simulink model "DIPCtranslation"  (R2014b)
settings: Solver=ode45  StartTime=0.0  StopTime=3.0  RelTol=1e-3
values from neighbouring files (symbols this model uses):
  deltav = 2000    [DIPCinit.m]
  ds = 0    [DIPCinit.m]
  dv = 5000    [DIPCinit.m]
  g = [0;0;0]    [DIPCinit.m]
  j0 = 1    [DIPCinit.m]
  j1 = 10    [DIPCinit.m]
  j2 = 10    [DIPCinit.m]
  j3 = 10    [DIPCinit.m]
  j4 = 10    [DIPCinit.m]
  jv = 1    [DIPCinit.m]
  kappav = 2000    [DIPCinit.m]
  ks = 3000    [DIPCinit.m]
  kv = 20000    [DIPCinit.m]
  m0 = 10    [DIPCinit.m]
  m1 = 10    [DIPCinit.m]
  m2 = 10    [DIPCinit.m]
  m3 = 10    [DIPCinit.m]
  m4 = 10    [DIPCinit.m]
  mv = 10    [DIPCinit.m]
libraries: aerolibutil x3, dspinverses x2, aerolibtransform2 x1, simulink x1
settings Model: Creator=Martin  LastModifiedBy=Martin

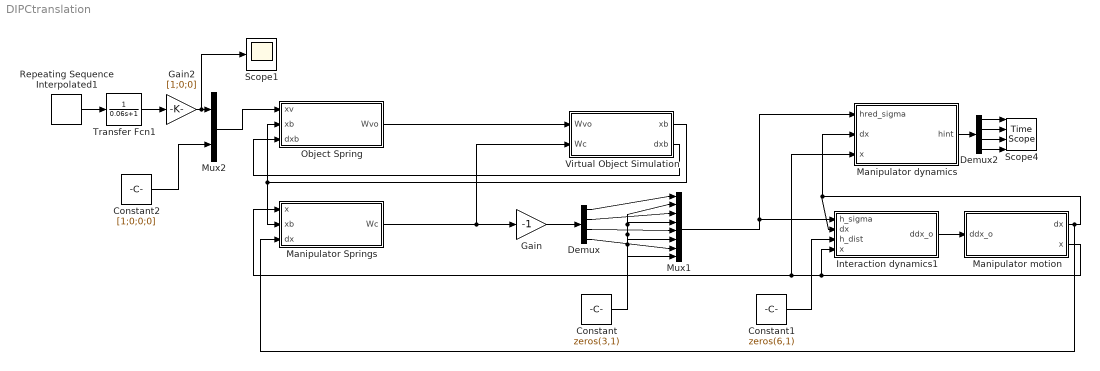
== system DIPCtranslation ==
  Constant : Constant  Value=zeros(3,1)
  Constant1 : Constant  Value=zeros(6,1)
  Constant2 : Constant  Value=[1;0;0;0]
  Demux : Demux
  Demux2 : Demux
  Gain : Gain  Gain=-1
  Gain2 : Gain  Gain=[1;0;0]
  Interaction dynamics1 : Subsystem
  Manipulator Springs : Subsystem
  Manipulator dynamics : Subsystem
  Manipulator motion : Subsystem
  Mux1 : Mux  Inputs=8
  Mux2 : Mux  Inputs=2
  Object Spring : Subsystem
  Repeating Sequence Interpolated1 : simulink/Sources/Repeating Sequence Interpolated  OutValues=[0 0 2 2 4 4 -2 -2 0 0].'  TimeValues=[0 0.1 0.14 0.9 0.96 1.8 1.95 2.4 2.6 3].'  LookUpMeth=Interpolation-Use End Values  tsamp=0.01  OutMin=[]  OutMax=[]  OutDataTypeStr=double  OutputDataTypeScalingMode=double  OutDataType=fixdt(0,8)  OutScaling=2^-10
  Scope1 : Scope
      settings: SaveName=ScopeData8
  Scope4 : TimeScope  NumInputPorts=4
  Transfer Fcn1 : TransferFcn  Denominator=[0.06 1]
  Virtual Object Simulation : Subsystem
  wires:
  Object Spring/1(Wvo) -> Virtual Object Simulation/1(Wvo)
  Virtual Object Simulation/1(xb) -> Object Spring/2(xb), Manipulator Springs/2(xb)
  Manipulator Springs/1(Wc) -> Gain/1, Virtual Object Simulation/2(Wc)
  Interaction dynamics1/1(ddx_o) -> Manipulator motion/1(ddx_o)
  Gain/1 -> Demux/1
  Demux/1 -> Mux1/1
  Demux/2 -> Mux1/3
  Constant/1 -> Mux1/8, Mux1/6, Mux1/4, Mux1/2
  Constant1/1 -> Interaction dynamics1/3(h_dist)
  Mux1/1 -> Manipulator dynamics/1(hred_sigma), Interaction dynamics1/1(h_sigma)
  Manipulator motion/1(dx) -> Manipulator Springs/3(dx), Manipulator dynamics/2(dx), Interaction dynamics1/2(dx)
  Manipulator motion/2(x) -> Manipulator dynamics/3(x), Manipulator Springs/1(x), Interaction dynamics1/4(x)
  Virtual Object Simulation/2(dxb) -> Object Spring/3(dxb)
  Demux/3 -> Mux1/5
  Demux/4 -> Mux1/7
  Manipulator dynamics/1(hint) -> Demux2/1
  Demux2/2 -> Scope4/2
  Demux2/4 -> Scope4/4
  Demux2/3 -> Scope4/3
  Demux2/1 -> Scope4/1
  Repeating Sequence Interpolated1/1 -> Transfer Fcn1/1
  Transfer Fcn1/1 -> Gain2/1
  Gain2/1 -> Scope1/1, Mux2/1
  Mux2/1 -> Object Spring/1(xv)
  Constant2/1 -> Mux2/2

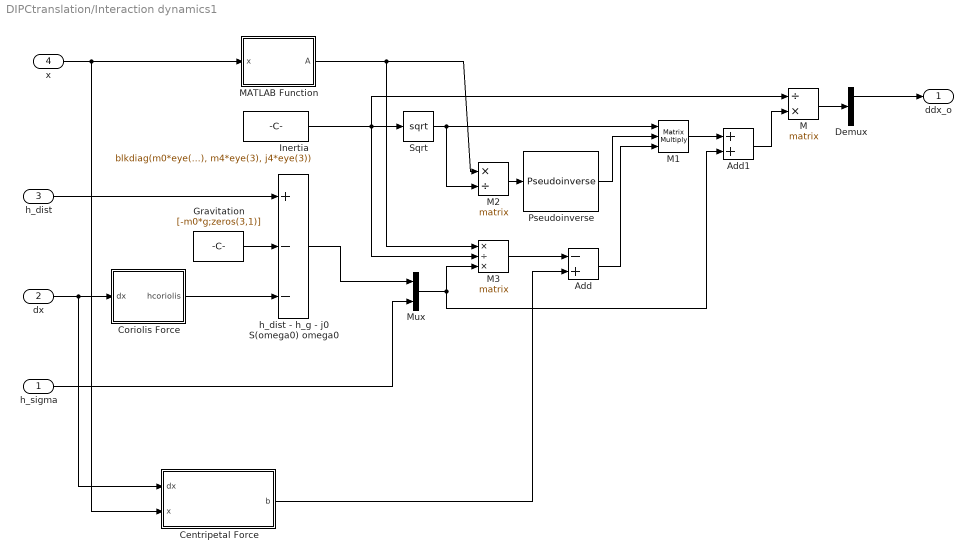
== system DIPCtranslation/Interaction dynamics1 ==
  h_sigma : Inport
  dx : Inport  Port=2
  h_dist : Inport  Port=3
  x : Inport  Port=4
  Add : Sum  Inputs=-+
  Add1 : Sum
  Centripetal Force : MATLAB Function  TreatAsAtomicUnit=on
  Coriolis Force : MATLAB Function  TreatAsAtomicUnit=on
  Demux : Demux  Outputs=5
  Gravitation : Constant  Value=[-m0*g;zeros(3,1)]
  Inertia : Constant  Value=blkdiag(m0*eye(3),j0*eye(3),m1*eye(3), j1*eye(3), m2*eye(3), j2*eye(3),m3*eye(3), j3*eye(3), m4*eye(3), j4*eye(3))
  M : Product  Inputs=/*  Multiplication=Matrix(*)
  M1 : Product  Inputs=***  Multiplication=Matrix(*)
  M2 : Product  Inputs=*/  Multiplication=Matrix(*)
  M3 : Product  Inputs=*/*  Multiplication=Matrix(*)
  MATLAB Function : MATLAB Function  TreatAsAtomicUnit=on
  Mux : Mux  Inputs=2
  Pseudoinverse : dspinverses/Pseudoinverse  wanterr=off
  Sqrt : Sqrt  SaturateOnIntegerOverflow=on
  "h_dist - h_g - j0 S(omega0) omega0 " : Sum  Inputs=+--
  ddx_o : Outport
  wires:
  h_dist/1 -> "h_dist - h_g - j0 S(omega0) omega0 "/1
  Gravitation/1 -> "h_dist - h_g - j0 S(omega0) omega0 "/2
  dx/1 -> Centripetal Force/1(dx), Coriolis Force/1(dx)
  Coriolis Force/1(hcoriolis) -> "h_dist - h_g - j0 S(omega0) omega0 "/3
  x/1 -> MATLAB Function/1(x), Centripetal Force/2(x)
  Inertia/1 -> M/1, M3/2, Sqrt/1
  Sqrt/1 -> M2/2, M1/1
  MATLAB Function/1(A) -> M3/1, M2/1
  M2/1 -> Pseudoinverse/1
  Pseudoinverse/1 -> M1/2
  Add/1 -> M1/3
  Centripetal Force/1(b) -> Add/2
  M3/1 -> Add/1
  Mux/1 -> Add1/2, M3/3
  "h_dist - h_g - j0 S(omega0) omega0 "/1 -> Mux/1
  h_sigma/1 -> Mux/2
  M/1 -> Demux/1
  Demux/1 -> ddx_o/1
  M1/1 -> Add1/1
  Add1/1 -> M/2

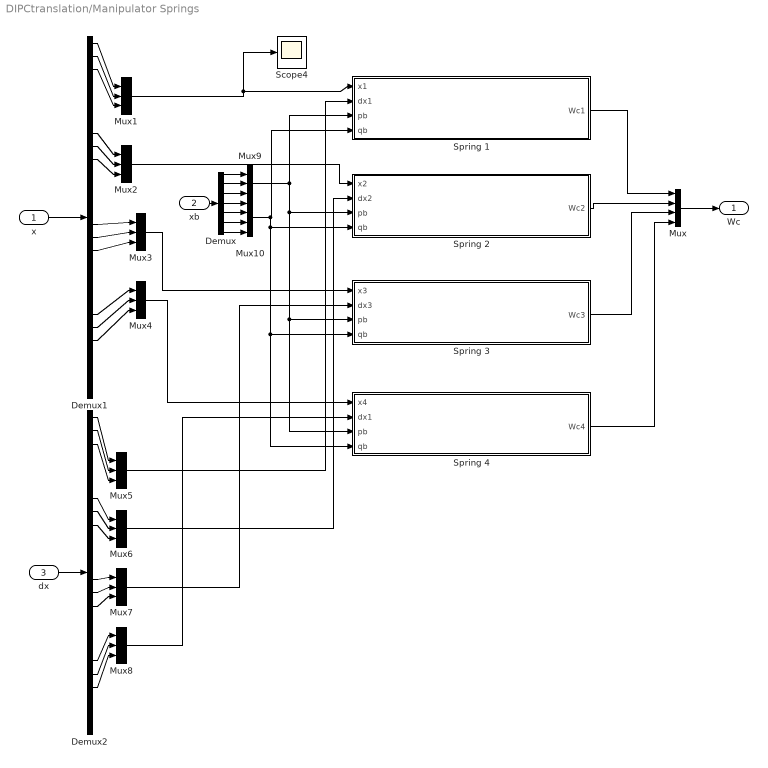
== system DIPCtranslation/Manipulator Springs ==
  x : Inport
  xb : Inport  Port=2
  dx : Inport  Port=3
  Demux : Demux  Outputs=7
  Demux1 : Demux  Outputs=28
  Demux2 : Demux  Outputs=24
  Mux : Mux
  Mux{1..9} (9 alike) : Mux  Inputs=3
  Mux10 : Mux
  Scope4 : Scope
      settings: SaveName=ScopeData2
  Spring 1 : Subsystem
  Spring 2 : Subsystem
  Spring 3 : Subsystem
  Spring 4 : Subsystem
  Wc : Outport
  wires:
  Spring 1/1(Wc1) -> Mux/1
  Spring 2/1(Wc2) -> Mux/2
  Mux/1 -> Wc/1
  x/1 -> Demux1/1
  Demux1/1 -> Mux1/1
  Demux1/2 -> Mux1/2
  Demux1/3 -> Mux1/3
  Demux1/8 -> Mux2/1
  Demux1/9 -> Mux2/2
  Demux1/10 -> Mux2/3
  Mux2/1 -> Spring 2/1(x2)
  Mux1/1 -> Scope4/1, Spring 1/1(x1)
  Spring 3/1(Wc3) -> Mux/3
  Spring 4/1(Wc4) -> Mux/4
  Demux1/15 -> Mux3/1
  Demux1/16 -> Mux3/2
  Demux1/17 -> Mux3/3
  Mux3/1 -> Spring 3/1(x3)
  Demux1/22 -> Mux4/1
  Demux1/23 -> Mux4/2
  Demux1/24 -> Mux4/3
  Mux4/1 -> Spring 4/1(x4)
  Demux2/1 -> Mux5/1
  Demux2/3 -> Mux5/3
  Demux2/2 -> Mux5/2
  Demux2/7 -> Mux6/1
  Demux2/8 -> Mux6/2
  Demux2/9 -> Mux6/3
  Demux2/13 -> Mux7/1
  Demux2/14 -> Mux7/2
  Demux2/15 -> Mux7/3
  Demux2/19 -> Mux8/1
  Demux2/20 -> Mux8/2
  Demux2/21 -> Mux8/3
  dx/1 -> Demux2/1
  Mux5/1 -> Spring 1/2(dx1)
  Mux6/1 -> Spring 2/2(dx2)
  Mux7/1 -> Spring 3/2(dx3)
  Mux8/1 -> Spring 4/2(dx1)
  xb/1 -> Demux/1
  Demux/1 -> Mux9/1
  Demux/2 -> Mux9/2
  Demux/3 -> Mux9/3
  Mux9/1 -> Spring 1/3(pb), Spring 2/3(pb), Spring 4/3(pb), Spring 3/3(pb)
  Demux/4 -> Mux10/1
  Demux/5 -> Mux10/2
  Demux/6 -> Mux10/3
  Demux/7 -> Mux10/4
  Mux10/1 -> Spring 4/4(qb), Spring 3/4(qb), Spring 2/4(qb), Spring 1/4(qb)

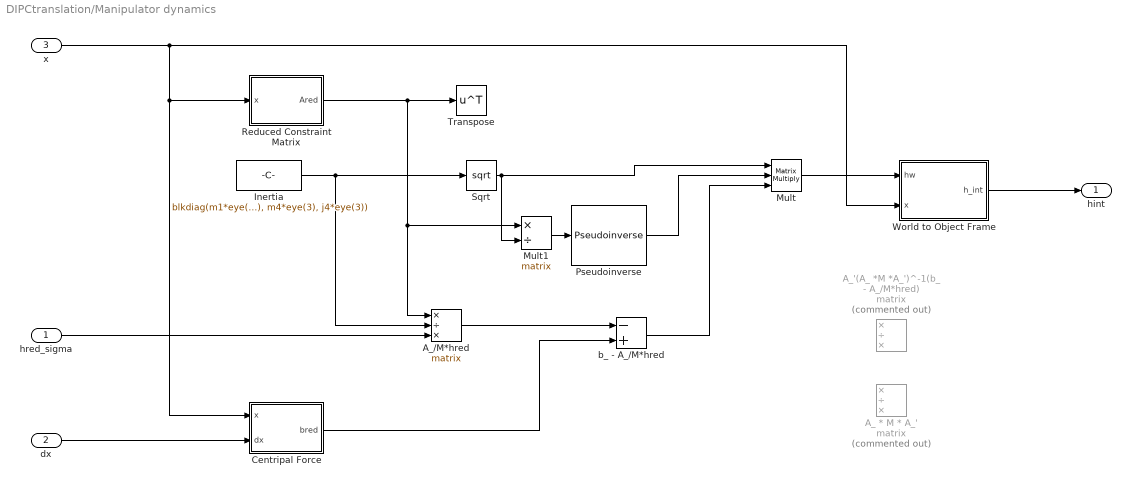
== system DIPCtranslation/Manipulator dynamics ==
  hred_sigma : Inport
  dx : Inport  Port=2
  x : Inport  Port=3
  A_ * M * A_' : Product  Commented=on  Inputs=*/*  Multiplication=Matrix(*)
  A_'(A_ *M *A_')^-1(b_ - A_/M*hred) : Product  Commented=on  Inputs=*/*  Multiplication=Matrix(*)
  A_/M*hred : Product  Inputs=*/*  Multiplication=Matrix(*)
  Centripal Force : MATLAB Function  TreatAsAtomicUnit=on
  Inertia : Constant  Value=blkdiag(m1*eye(3), j1*eye(3), m2*eye(3), j2*eye(3), m3*eye(3), j3*eye(3), m4*eye(3), j4*eye(3))
  Mult : Product  Inputs=***  Multiplication=Matrix(*)
  Mult1 : Product  Inputs=*/  Multiplication=Matrix(*)
  Pseudoinverse : dspinverses/Pseudoinverse  wanterr=off
  Reduced Constraint Matrix : MATLAB Function  TreatAsAtomicUnit=on
  Sqrt : Sqrt  SaturateOnIntegerOverflow=on
  Transpose : Math  Operator=transpose  SaturateOnIntegerOverflow=on
  World to Object Frame : MATLAB Function  TreatAsAtomicUnit=on
  b_ - A_/M*hred : Sum  Inputs=-+
  hint : Outport
  wires:
  Reduced Constraint Matrix/1(Ared) -> Transpose/1, A_/M*hred/1, Mult1/1
  Inertia/1 -> Sqrt/1, A_/M*hred/2
  dx/1 -> Centripal Force/2(dx)
  A_/M*hred/1 -> b_ - A_/M*hred/1
  hred_sigma/1 -> A_/M*hred/3
  World to Object Frame/1(h_int) -> hint/1
  x/1 -> Centripal Force/1(x), Reduced Constraint Matrix/1(x), World to Object Frame/2(x)
  Centripal Force/1(bred) -> b_ - A_/M*hred/2
  Mult/1 -> World to Object Frame/1(hw)
  b_ - A_/M*hred/1 -> Mult/3
  Sqrt/1 -> Mult1/2, Mult/1
  Mult1/1 -> Pseudoinverse/1
  Pseudoinverse/1 -> Mult/2

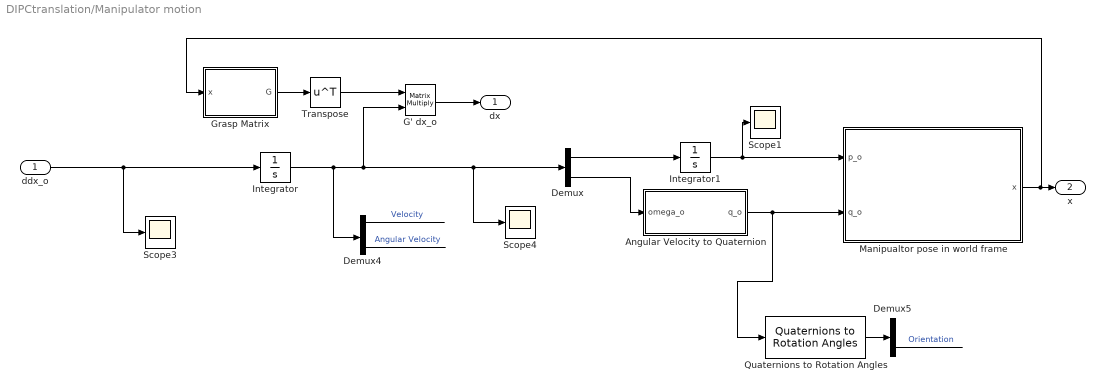
== system DIPCtranslation/Manipulator motion ==
  ddx_o : Inport
  Angular Velocity to Quaternion : Subsystem
  Demux : Demux  Outputs=2
  Demux4 : Demux  Outputs=6
  Demux5 : Demux  Outputs=3
  G' dx_o : Product  Multiplication=Matrix(*)
  Grasp Matrix : MATLAB Function  TreatAsAtomicUnit=on
  Integrator : Integrator  InitialCondition=zeros(6,1)
  Integrator1 : Integrator  InitialCondition=[0 0 0]'
  Manipualtor pose in world frame : MATLAB Function  TreatAsAtomicUnit=on
  Quaternions to Rotation Angles : aerolibtransform2/Quaternions to Rotation Angles  rotationOrder=XYZ
  Scope1 : Scope
  Scope3 : Scope
      settings: SaveName=ScopeData7
  Scope4 : Scope
      settings: SaveName=ScopeData16
  Transpose : Math  Operator=transpose  SaturateOnIntegerOverflow=on
  dx : Outport
  x : Outport  Port=2
  wires:
  ddx_o/1 -> Scope3/1, Integrator/1
  Integrator/1 -> Demux4/1, G' dx_o/2, Scope4/1, Demux/1
  Grasp Matrix/1(G) -> Transpose/1
  Transpose/1 -> G' dx_o/1
  G' dx_o/1 -> dx/1
  Demux/2 -> Angular Velocity to Quaternion/1(omega_o)
  Demux/1 -> Integrator1/1
  Integrator1/1 -> Scope1/1, Manipualtor pose in world frame/1(p_o)
  Manipualtor pose in world frame/1(x) -> Grasp Matrix/1(x), x/1
  Angular Velocity to Quaternion/1(q_o) -> Quaternions to Rotation Angles/1, Manipualtor pose in world frame/2(q_o)
  Demux4/1 -> ?  "Velocity"
  Demux4/6 -> ?  "Angular Velocity"
  Quaternions to Rotation Angles/1 -> Demux5/1
  Demux5/3 -> ?  "Orientation"

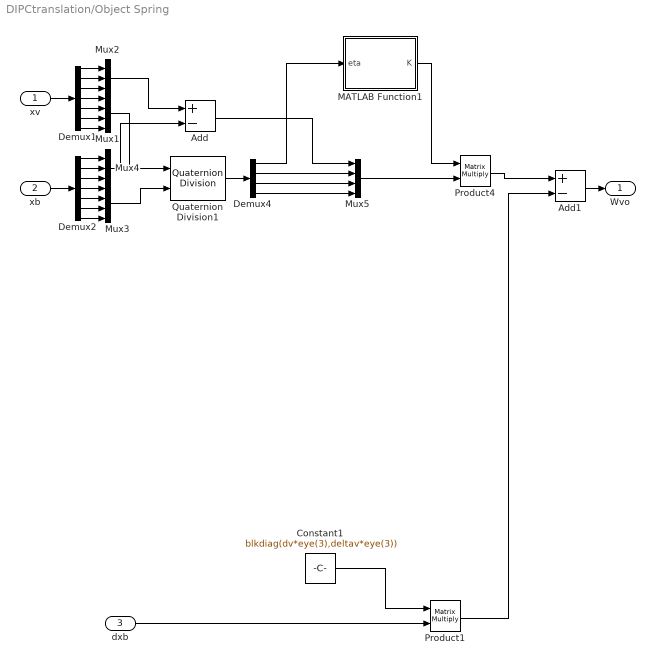
== system DIPCtranslation/Object Spring ==
  xv : Inport
  xb : Inport  Port=2
  dxb : Inport  Port=3
  Add : Sum  Inputs=+-
  Add1 : Sum  Inputs=+-
  Constant1 : Constant  Value=blkdiag(dv*eye(3),deltav*eye(3))
  Demux1 : Demux  Outputs=7
  Demux2 : Demux  Outputs=7
  Demux4 : Demux
  MATLAB Function1 : MATLAB Function  TreatAsAtomicUnit=on
  Mux1 : Mux
  Mux2 : Mux  Inputs=3
  Mux3 : Mux
  Mux4 : Mux  Inputs=3
  Mux5 : Mux
  Product1 : Product  Multiplication=Matrix(*)
  Product4 : Product  Multiplication=Matrix(*)
  Quaternion Division1 : aerolibutil/Quaternion Division
  Wvo : Outport
  wires:
  Add1/1 -> Wvo/1
  Product4/1 -> Add1/1
  Product1/1 -> Add1/2
  dxb/1 -> Product1/2
  Constant1/1 -> Product1/1
  MATLAB Function1/1(K) -> Product4/1
  Demux4/1 -> MATLAB Function1/1(eta)
  Add/1 -> Mux5/1
  Demux4/2 -> Mux5/2
  Demux4/3 -> Mux5/3
  Demux4/4 -> Mux5/4
  Quaternion Division1/1 -> Demux4/1
  Mux5/1 -> Product4/2
  xv/1 -> Demux1/1
  xb/1 -> Demux2/1
  Demux1/4 -> Mux1/1
  Demux1/5 -> Mux1/2
  Demux1/6 -> Mux1/3
  Demux1/7 -> Mux1/4
  Demux1/1 -> Mux2/1
  Demux1/2 -> Mux2/2
  Demux1/3 -> Mux2/3
  Mux2/1 -> Add/1
  Mux1/1 -> Quaternion Division1/1
  Demux2/4 -> Mux3/1
  Demux2/5 -> Mux3/2
  Demux2/6 -> Mux3/3
  Demux2/7 -> Mux3/4
  Demux2/1 -> Mux4/1
  Demux2/2 -> Mux4/2
  Demux2/3 -> Mux4/3
  Mux4/1 -> Add/2
  Mux3/1 -> Quaternion Division1/2

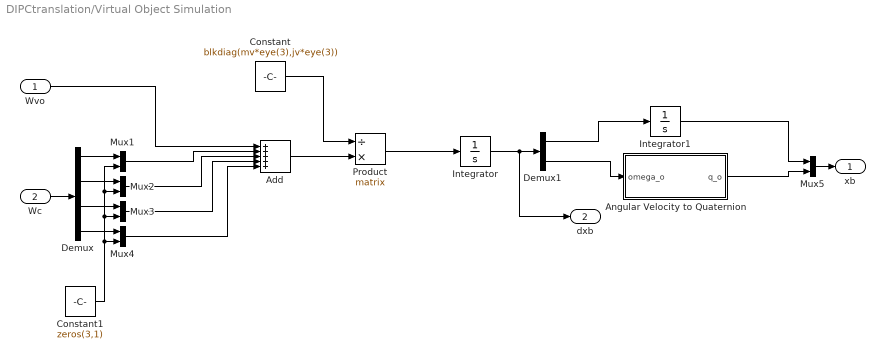
== system DIPCtranslation/Virtual Object Simulation ==
  Wvo : Inport
  Wc : Inport  Port=2
  Add : Sum  Inputs=+++++
  Angular Velocity to Quaternion : Subsystem
  Constant : Constant  Value=blkdiag(mv*eye(3),jv*eye(3))
  Constant1 : Constant  Value=zeros(3,1)
  Demux : Demux
  Demux1 : Demux  Outputs=2
  Integrator : Integrator  InitialCondition=zeros(6,1)
  Integrator1 : Integrator  InitialCondition=[0 0 0]'
  Mux{1..5} (5 alike) : Mux  Inputs=2
  Product : Product  Inputs=/*  Multiplication=Matrix(*)
  xb : Outport
  dxb : Outport  Port=2
  wires:
  Wc/1 -> Demux/1
  Wvo/1 -> Add/1
  Add/1 -> Product/2
  Constant/1 -> Product/1
  Product/1 -> Integrator/1
  Integrator/1 -> Demux1/1, dxb/1
  Demux/1 -> Mux1/1
  Demux/4 -> Mux4/1
  Demux/3 -> Mux3/1
  Demux/2 -> Mux2/1
  Constant1/1 -> Mux4/2, Mux3/2, Mux2/2, Mux1/2
  Mux1/1 -> Add/2
  Mux2/1 -> Add/3
  Mux3/1 -> Add/4
  Mux4/1 -> Add/5
  Demux1/2 -> Angular Velocity to Quaternion/1(omega_o)
  Demux1/1 -> Integrator1/1
  Integrator1/1 -> Mux5/1
  Angular Velocity to Quaternion/1(q_o) -> Mux5/2
  Mux5/1 -> xb/1

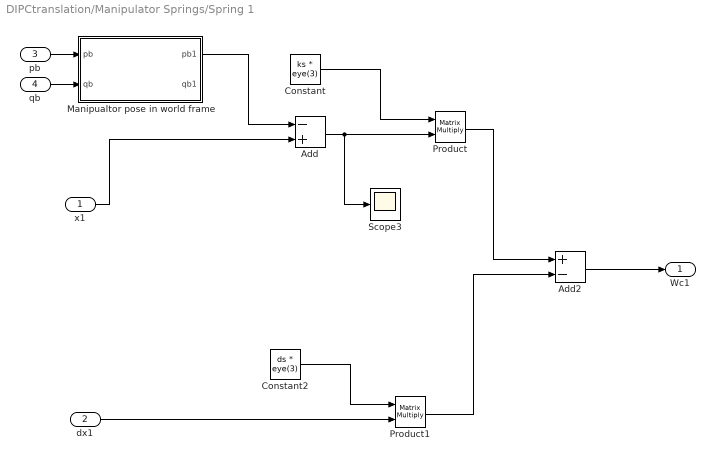
== system DIPCtranslation/Manipulator Springs/Spring 1 ==
  x1 : Inport
  dx1 : Inport  Port=2
  pb : Inport  Port=3
  qb : Inport  Port=4
  Add : Sum  Inputs=-+
  Add2 : Sum  Inputs=+-
  Constant : Constant  Value=ks * eye(3)
  Constant2 : Constant  Value=ds * eye(3)
  Manipualtor pose in world frame : MATLAB Function  TreatAsAtomicUnit=on
  Product : Product  Multiplication=Matrix(*)
  Product1 : Product  Multiplication=Matrix(*)
  Scope3 : Scope
      settings: SaveName=ScopeData5
  Wc1 : Outport
  wires:
  x1/1 -> Add/2
  Add/1 -> Scope3/1, Product/2
  Constant/1 -> Product/1
  Product1/1 -> Add2/2
  dx1/1 -> Product1/2
  Constant2/1 -> Product1/1
  Add2/1 -> Wc1/1
  Product/1 -> Add2/1
  pb/1 -> Manipualtor pose in world frame/1(pb)
  qb/1 -> Manipualtor pose in world frame/2(qb)
  Manipualtor pose in world frame/1(pb1) -> Add/1

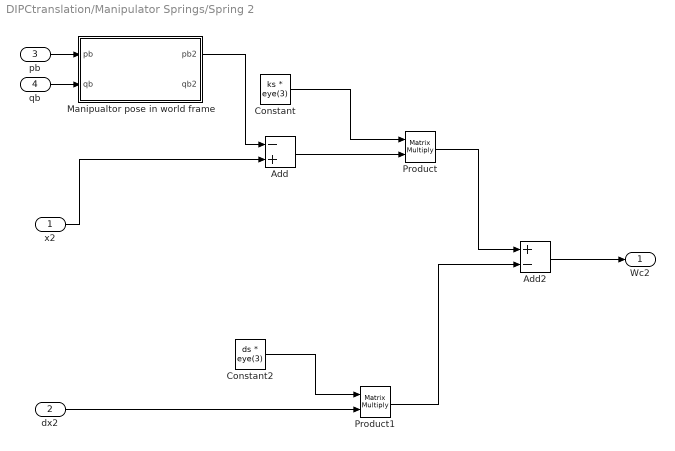
== system DIPCtranslation/Manipulator Springs/Spring 2 ==
  x2 : Inport
  dx2 : Inport  Port=2
  pb : Inport  Port=3
  qb : Inport  Port=4
  Add : Sum  Inputs=-+
  Add2 : Sum  Inputs=+-
  Constant : Constant  Value=ks * eye(3)
  Constant2 : Constant  Value=ds * eye(3)
  Manipualtor pose in world frame : MATLAB Function  TreatAsAtomicUnit=on
  Product : Product  Multiplication=Matrix(*)
  Product1 : Product  Multiplication=Matrix(*)
  Wc2 : Outport
  wires:
  x2/1 -> Add/2
  Add/1 -> Product/2
  Constant/1 -> Product/1
  Product1/1 -> Add2/2
  dx2/1 -> Product1/2
  Constant2/1 -> Product1/1
  Add2/1 -> Wc2/1
  Product/1 -> Add2/1
  pb/1 -> Manipualtor pose in world frame/1(pb)
  qb/1 -> Manipualtor pose in world frame/2(qb)
  Manipualtor pose in world frame/1(pb2) -> Add/1

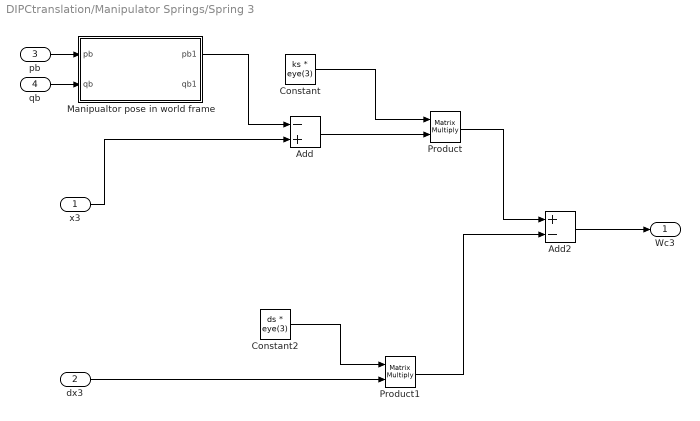
== system DIPCtranslation/Manipulator Springs/Spring 3 ==
  x3 : Inport
  dx3 : Inport  Port=2
  pb : Inport  Port=3
  qb : Inport  Port=4
  Add : Sum  Inputs=-+
  Add2 : Sum  Inputs=+-
  Constant : Constant  Value=ks * eye(3)
  Constant2 : Constant  Value=ds * eye(3)
  Manipualtor pose in world frame : MATLAB Function  TreatAsAtomicUnit=on
  Product : Product  Multiplication=Matrix(*)
  Product1 : Product  Multiplication=Matrix(*)
  Wc3 : Outport
  wires:
  x3/1 -> Add/2
  Add/1 -> Product/2
  Constant/1 -> Product/1
  Product1/1 -> Add2/2
  dx3/1 -> Product1/2
  Constant2/1 -> Product1/1
  Add2/1 -> Wc3/1
  Product/1 -> Add2/1
  pb/1 -> Manipualtor pose in world frame/1(pb)
  qb/1 -> Manipualtor pose in world frame/2(qb)
  Manipualtor pose in world frame/1(pb1) -> Add/1

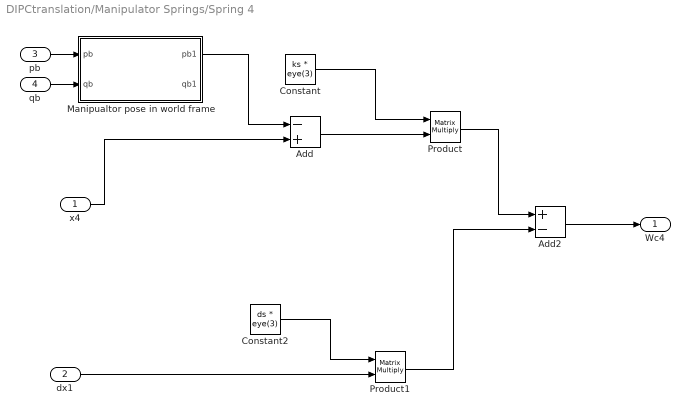
== system DIPCtranslation/Manipulator Springs/Spring 4 ==
  x4 : Inport
  dx1 : Inport  Port=2
  pb : Inport  Port=3
  qb : Inport  Port=4
  Add : Sum  Inputs=-+
  Add2 : Sum  Inputs=+-
  Constant : Constant  Value=ks * eye(3)
  Constant2 : Constant  Value=ds * eye(3)
  Manipualtor pose in world frame : MATLAB Function  TreatAsAtomicUnit=on
  Product : Product  Multiplication=Matrix(*)
  Product1 : Product  Multiplication=Matrix(*)
  Wc4 : Outport
  wires:
  x4/1 -> Add/2
  Add/1 -> Product/2
  Constant/1 -> Product/1
  Product1/1 -> Add2/2
  dx1/1 -> Product1/2
  Constant2/1 -> Product1/1
  Add2/1 -> Wc4/1
  Product/1 -> Add2/1
  pb/1 -> Manipualtor pose in world frame/1(pb)
  qb/1 -> Manipualtor pose in world frame/2(qb)
  Manipualtor pose in world frame/1(pb1) -> Add/1

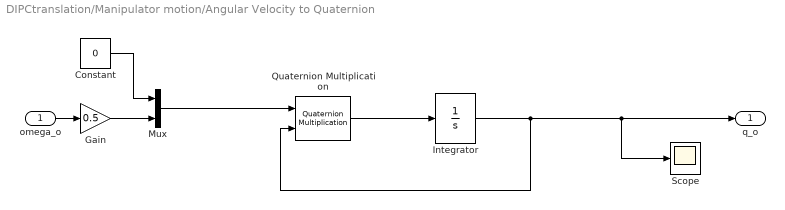
== system DIPCtranslation/Manipulator motion/Angular Velocity to Quaternion ==
  omega_o : Inport
  Constant : Constant  Value=0
  Gain : Gain  Gain=0.5
  Integrator : Integrator  InitialCondition=[1; 0; 0; 0]
  Mux : Mux  Inputs=2
  Quaternion Multiplication : aerolibutil/Quaternion Multiplication
  Scope : Scope
      settings: ShowLegends=on  SaveName=ScopeData9
  q_o : Outport
  wires:
  omega_o/1 -> Gain/1
  Gain/1 -> Mux/2
  Constant/1 -> Mux/1
  Quaternion Multiplication/1 -> Integrator/1
  Integrator/1 -> Quaternion Multiplication/2, q_o/1, Scope/1
  Mux/1 -> Quaternion Multiplication/1

== system DIPCtranslation/Virtual Object Simulation/Angular Velocity to Quaternion ==
  omega_o : Inport
  Constant : Constant  Value=0
  Gain : Gain  Gain=0.5
  Integrator : Integrator  InitialCondition=[1; 0; 0; 0]
  Mux : Mux  Inputs=2
  Quaternion Multiplication : aerolibutil/Quaternion Multiplication
  Scope : Scope
      settings: ShowLegends=on  SaveName=ScopeData9
  q_o : Outport
  wires:
  omega_o/1 -> Gain/1
  Gain/1 -> Mux/2
  Constant/1 -> Mux/1
  Quaternion Multiplication/1 -> Integrator/1
  Integrator/1 -> Quaternion Multiplication/2, q_o/1, Scope/1
  Mux/1 -> Quaternion Multiplication/1

== matlab function DIPCtranslation/Manipulator Springs/Spring 1/Manipualtor pose in world frame ==
  data: pb input; qb input size=4; pb1 output; r parameter; qb1 output
function [pb1,qb1]= manipulatorpose(pb,qb,r)

pb1 = pb + quatrot(qb,r(1:3));
qb1 = qb;

== matlab function DIPCtranslation/Manipulator Springs/Spring 2/Manipualtor pose in world frame ==
  data: pb input; qb input size=4; pb2 output; r parameter; qb2 output
function [pb2,qb2]= manipulatorpose(pb,qb,r)

pb2 = pb + quatrot(qb,r(4:6));
qb2 = qb;

== matlab function DIPCtranslation/Manipulator Springs/Spring 3/Manipualtor pose in world frame ==
  data: pb input; qb input size=4; pb1 output; r parameter; qb1 output
function [pb1,qb1]= manipulatorpose(pb,qb,r)

pb1 = pb + quatrot(qb,r(7:9));
qb1 = qb;

== matlab function DIPCtranslation/Manipulator Springs/Spring 4/Manipualtor pose in world frame ==
  data: pb input; qb input size=4; pb1 output; r parameter; qb1 output
function [pb1,qb1]= manipulatorpose(pb,qb,r)

pb1 = pb + quatrot(qb,r(10:12));
qb1 = qb;

== matlab function DIPCtranslation/Interaction dynamics1/MATLAB Function ==
  data: r parameter; A output; x input
function A = ConstraintMatrix(r,x)
A = [-eye(3) skew_sm(quatrot(x(4:7),r(1:3))) eye(3) zeros(3,21);
        zeros(3) -eye(3) zeros(3) eye(3) zeros(3,18);
        -eye(3) skew_sm(quatrot(x(4:7),r(4:6))) zeros(3,6) eye(3) zeros(3,15);
        zeros(3) -eye(3) zeros(3,9) eye(3) zeros(3,12);
        -eye(3) skew_sm(quatrot(x(4:7),r(7:9))) zeros(3,12) eye(3) zeros(3,9);
        zeros(3) -eye(3) zeros(3,15) eye(3) zeros(3,6);
        -eye(3) skew_sm(quatrot(x(4:7),r(10:12))) zeros(3,18) eye(3) zeros(3);
        zeros(3) -eye(3) zeros(3,21) eye(3)];

== matlab function DIPCtranslation/Interaction dynamics1/Centripetal Force ==
  data: dx input; b output; r parameter; x input
function b = centripetalforce(dx,r,x)
b = [skew_sm(dx(4:6))*skew_sm(dx(4:6))*quatrot(x(4:7),r(1:3));
     zeros(3,1);
     skew_sm(dx(4:6))*skew_sm(dx(4:6))*quatrot(x(4:7),r(4:6));
     zeros(3,1);
     skew_sm(dx(4:6))*skew_sm(dx(4:6))*quatrot(x(4:7),r(7:9));
     zeros(3,1);
     skew_sm(dx(4:6))*skew_sm(dx(4:6))*quatrot(x(4:7),r(10:12));
     zeros(3,1)];

== matlab function DIPCtranslation/Interaction dynamics1/Coriolis Force ==
  data: dx input; hcoriolis output; j0 parameter; m0 parameter
function hcoriolis = CoriolisForce(dx,j0,m0)
hcoriolis = [m0*skew_sm(dx(4:6))*dx(1:3);
        j0*skew_sm(dx(4:6))*dx(4:6)];

== matlab function DIPCtranslation/Object Spring/MATLAB Function1 ==
  data: eta input; K output; kv parameter; kappav parameter
function K = stiffness(eta,kv,kappav)
K = blkdiag(kv*eye(3),2*eta*kappav*eye(3));

== matlab function DIPCtranslation/Manipulator dynamics/Reduced Constraint Matrix ==
  data: r parameter; Ared output; x input
function Ared = ReducedConstraintMAtrix(r,x)
Ared = [-eye(3) skew_sm(quatrot(x(4:7),r(4:6)-r(1:3))) eye(3) zeros(3,15);
        zeros(3) -eye(3) zeros(3) eye(3) zeros(3,12);
        -eye(3) skew_sm(quatrot(x(4:7),r(7:9)-r(1:3))) zeros(3,6) eye(3) zeros(3,9);
        zeros(3) -eye(3) zeros(3,9) eye(3) zeros(3,6);
        -eye(3) skew_sm(quatrot(x(4:7),r(10:12)-r(1:3))) zeros(3,12) eye(3) zeros(3);
        zeros(3) -eye(3) zeros(3,15) eye(3)];

== matlab function DIPCtranslation/Manipulator dynamics/Centripal Force ==
  data: r parameter; x input; bred output; dx input
function bred = ReducedCentripetalvector(r,x,dx)
bred = [skew_sm(dx(4:6))*skew_sm(dx(4:6))*quatrot(x(4:7),(r(4:6)-r(1:3)));
        zeros(3,1);
        skew_sm(dx(4:6))*skew_sm(dx(4:6))*quatrot(x(4:7),(r(7:9)-r(1:3)));
        zeros(3,1);
        skew_sm(dx(4:6))*skew_sm(dx(4:6))*quatrot(x(4:7),(r(10:12)-r(1:3)));
        zeros(3,1)];

== matlab function DIPCtranslation/Manipulator motion/Grasp Matrix ==
  data: r parameter; G output; x input
function G = GraspMatrix(r,x)
G = [eye(3) zeros(3) eye(3) zeros(3) eye(3) zeros(3) eye(3) zeros(3);
    skew_sm(quatrot(x(4:7),r(1:3))) eye(3) skew_sm(quatrot(x(4:7),r(4:6))) eye(3) skew_sm(quatrot(x(4:7),r(7:9))) eye(3) skew_sm(quatrot(x(4:7),r(10:12))) eye(3)];

== matlab function DIPCtranslation/Manipulator motion/Manipualtor pose in world frame ==
  data: p_o input; q_o input size=4; x output; r parameter
function x = manipulatorpose(p_o,q_o,r)

x = [p_o + quatrot(q_o,r(1:3));
        q_o;
        p_o + quatrot(q_o,r(4:6));
        q_o;
        p_o + quatrot(q_o,r(7:9));
        q_o;
        p_o + quatrot(q_o,r(10:12));
        q_o ];

== matlab function DIPCtranslation/Manipulator dynamics/World to Object Frame ==
  data: hw input; x input; h_int output
function h_int = inertial2objectFrame(hw,x)

h_int = [quatrot(quatconj(x(4:7)')',hw(1:3));
         hw(4:6);%quatrot(quatconj(x(4:7)')',hw(4:6));
         quatrot(quatconj(x(4:7)')',hw(7:9));
         hw(10:12);%quatrot(quatconj(x(4:7)')',hw(10:12));
         quatrot(quatconj(x(4:7)')',hw(13:15));
         hw(16:18);%quatrot(quatconj(x(4:7)')',hw(16:18));
         quatrot(quatconj(x(4:7)')',hw(19:21));
         hw(22:24)];%quatrot(quatconj(x(4:7)')',hw(22:24));];
